simulink model "lab7"  (R2015a)
settings: Solver=ode45  StartTime=0.0  StopTime=390  RelTol=1e-3
undefined symbols (not defined in the file or in its folder): currentCFG_lab7_UB, fdesignblkfcn, gcbh, UB
libraries: dspstat3 x2, gtecHighspeedLib x1, gUSBamplib x1
settings Model: Creator=circuit  LastModifiedBy=circuit

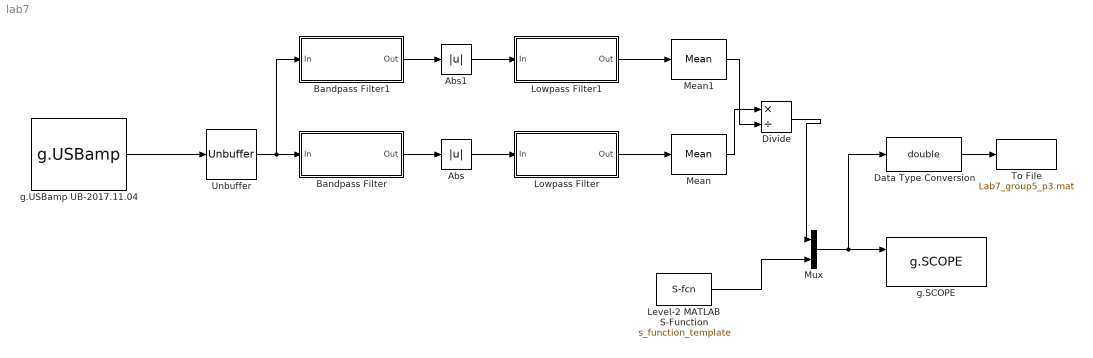
== system lab7 ==
  Abs : Abs
  Abs1 : Abs
  Bandpass Filter : Subsystem  DialogController=fdesignblkfcn  InitFcn=fdesignblkfcn(gcbh, {'InitFcn'});  mask(Bandpass Filter){}
      mask help: Design a bandpass filter
      settings: CopyFcn=fdesignblkfcn(gcbh, {'CopyFcn'});
      mask Help: helpview(mapfilelocation('dsp'), 'dspbandpassfilter');
      mask Display: disp('Bandpass');
  Bandpass Filter1 : Subsystem  DialogController=fdesignblkfcn  InitFcn=fdesignblkfcn(gcbh, {'InitFcn'});  mask(Bandpass Filter){}
      mask help: Design a bandpass filter
      settings: CopyFcn=fdesignblkfcn(gcbh, {'CopyFcn'});
      mask Help: helpview(mapfilelocation('dsp'), 'dspbandpassfilter');
      mask Display: disp('Bandpass');
  Data Type Conversion : DataTypeConversion  OutDataTypeStr=double
  Divide : Product  Inputs=*/
  Level-2 MATLAB S-Function : M-S-Function  FunctionName=s_function_template
  Lowpass Filter : Subsystem  DialogController=fdesignblkfcn  InitFcn=fdesignblkfcn(gcbh, {'InitFcn'});  mask(Lowpass Filter){}
      mask help: Design a lowpass filter
      settings: CopyFcn=fdesignblkfcn(gcbh, {'CopyFcn'});
      mask Help: helpview(mapfilelocation('dsp'), 'dsplowpassfilter');
      mask Display: disp('Lowpass')
  Lowpass Filter1 : Subsystem  DialogController=fdesignblkfcn  InitFcn=fdesignblkfcn(gcbh, {'InitFcn'});  mask(Lowpass Filter){}
      mask help: Design a lowpass filter
      settings: CopyFcn=fdesignblkfcn(gcbh, {'CopyFcn'});
      mask Help: helpview(mapfilelocation('dsp'), 'dsplowpassfilter');
      mask Display: disp('Lowpass')
  Mean : dspstat3/Mean  run=off  reset_popup=None  InputProcessing=Columns as channels (frame based)  directionMode=Each row  dimension=1  treatSBRowAsCol=off  roiEnable=off  roiType=Rectangles  roiPortion=Entire ROI  roiOutput=Individual statistics for each ROI  roiFlag=off  outputDataTypeStr=Inherit: Same as accumulator  outputLastDataTypeStr=Inherit: Same as accumulator  outputMin=[]  outputMax=[]  roundingMode=Floor  overflowMode=off
  Mean1 : dspstat3/Mean  run=off  reset_popup=None  InputProcessing=Columns as channels (frame based)  directionMode=Each row  dimension=1  treatSBRowAsCol=off  roiEnable=off  roiType=Rectangles  roiPortion=Entire ROI  roiOutput=Individual statistics for each ROI  roiFlag=off  outputDataTypeStr=Inherit: Same as accumulator  outputLastDataTypeStr=Inherit: Same as accumulator  outputMin=[]  outputMax=[]  roundingMode=Floor  overflowMode=off
  Mux : Mux  Inputs=2
  To File : ToFile  Filename=Lab7_group5_p3.mat
  Unbuffer : Unbuffer  SampleBasedProcessing=Same as frame based
  g.SCOPE : gtecHighspeedLib/g.SCOPE
  g.USBamp UB-2017.11.04 : gUSBamplib/g.USBamp  cfg=currentCFG_lab7_UB-2017.11.04.cfg  snr=UB-2017.11.04
  wires:
  g.USBamp UB-2017.11.04/1 -> Unbuffer/1
  Bandpass Filter/1(Out) -> Abs/1
  Abs/1 -> Lowpass Filter/1(In)
  Lowpass Filter/1(Out) -> Mean/1
  Unbuffer/1 -> Bandpass Filter1/1(In), Bandpass Filter/1(In)
  Mux/1 -> Data Type Conversion/1, g.SCOPE/1
  Level-2 MATLAB S-Function/1 -> Mux/2
  Data Type Conversion/1 -> To File/1
  Bandpass Filter1/1(Out) -> Abs1/1
  Abs1/1 -> Lowpass Filter1/1(In)
  Lowpass Filter1/1(Out) -> Mean1/1
  Mean/1 -> Divide/1
  Mean1/1 -> Divide/2
  Divide/1 -> Mux/1

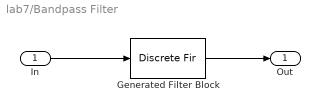
== system lab7/Bandpass Filter ==
  In : Inport
  Generated Filter Block : DiscreteFir  Tag=BlockMethodSubSystem  Coefficients=[2.7190426698472572e-18 -1.0908185879633193e-05 1.520684445102344e-05 5.9315566798347776e-05 5.800034854108737e-05 -2.0396570865799991e-05 -0.00011845969573629914 -0.00012738266702765806 -1.1513153684603061e-19 0.00017272582002327323 0.00021950102083968773 5.2546096976351294e-05 -0.00021434299056270176 -0.00033253314769670164 -0.00014434765399001844 0.0002320364222776027 0.00046047217716153568 0.00028094492726581474 -0.00021174425558163697 -0.00059175018646499215 -0.00046367795469145871 0.00013860058094126063 0.00070895386584620811 0.00068712060084153684 -2.0074243731143294e-18 -0.00079002026862442284 -0.00093727551956054834 -0.00021073549795040954 0.00081102828190988692 0.0011911833363798426 0.00049080070902079618 -0.00075036401862936866 -0.0014184160470135699 -0.00082529572189400115 0.00059369534792681842 0.001584616182718924 0.0011863604619702602 -0.00033890853760402013 -0.001656854224615913 -0.0015346613168919863 -3.7476367741136453e-18 0.0016101709367714611 0.0018234925555774587 0.00039107627928343391 -0.0014343221416268494 -0.0020053091123723812 -0.00078541019388994712 0.001139521741680656 0.002040026188317274 0.0011214198244585052 -0.00075994002810688712 -0.0019039859739218034 -0.001332349683241074 0.00035388793624190003 0.0015981839151395199 0.0013563494031183791 -1.167034324091124e-18 -0.0011542342098058455 -0.0011479613184324207 -0.00021072008592950235 0.00063667861703461156 0.00068942638733922442 0.00018647850248215282 -0.0001406111708457172 -1.8353538021468985e-17 0.00015127026108370566 -0.00021582800879737016 -0.00085849027561536707 -0.00085304304480034567 0.00030381291102699509 0.0017812926009562861 0.0019278780158680892 -1.6322403253386542e-18 -0.002626452444663831 -0.0033333696475308394 -0.00079524173104250531 0.0032266997021166946 0.0049711137239133365 0.002139805193973388 -0.0034067185066119035 -0.0066889508236326707 -0.0040345346627025658 0.0030041643873728783 0.0082906046554809907 0.0064130493527291259 -0.0018920899597823313 -0.0095523575352329977 -0.0091386778220399634 -2.4057070663414456e-18 0.010245413307559797 0.0120097217529452 0.0026693368020745799 -0.010161706291930863 -0.014773277235232266 -0.0060298998785369004 0.0091402560631568073 0.017146741075987779 0.0099111688340985694 -0.0070908496363779249 -0.018845064066358108 -0.014066562886420964 0.0040119204928050064 0.019610930916622103 0.018191355541196143 -2.0721869535670114e-17 -0.019244478222364952 -0.021948648476352237 -0.0047510042785245737 0.017629000615502922 0.025000899763098283 0.0099612960891193574 -0.014749382546861711 -0.027043678172353688 -0.015286750482589083 0.01070071066686748 0.027837877532802983 0.020348597794259786 -0.0056855921470147308 -0.02723664502279062 -0.024768224255709254 0 0.025203767584335721 0.028203363377651062 0.0059911738926469475 -0.02182117135681989 -0.030381676304823767 -0.011886427654215447 0.017284412946531557 0.031127931526122532 0.017284412946531557 -0.011886427654215447 -0.030381676304823767 -0.02182117135681989 0.0059911738926469475 0.028203363377651062 0.025203767584335721 0 -0.024768224255709254 -0.02723664502279062 -0.0056855921470147308 0.020348597794259786 0.027837877532802983 0.01070071066686748 -0.015286750482589083 -0.027043678172353688 -0.014749382546861711 0.0099612960891193574 0.025000899763098283 0.017629000615502922 -0.0047510042785245737 -0.021948648476352237 -0.019244478222364952 -2.0721869535670114e-17 0.018191355541196143 0.019610930916622103 0.0040119204928050064 -0.014066562886420964 -0.018845064066358108 -0.0070908496363779249 0.0099111688340985694 0.017146741075987779 0.0091402560631568073 -0.0060298998785369004 -0.014773277235232266 -0.010161706291930863 0.0026693368020745799 0.0120097217529452 0.010245413307559797 -2.4057070663414456e-18 -0.0091386778220399634 -0.0095523575352329977 -0.0018920899597823313 0.0064130493527291259 0.0082906046554809907 0.0030041643873728783 -0.0040345346627025658 -0.0066889508236326707 -0.0034067185066119035 0.002139805193973388 0.0049711137239133365 ...(+1777 chars)]  InputProcessing=Columns as channels (frame based)
  Out : Outport
  wires:
  In/1 -> Generated Filter Block/1
  Generated Filter Block/1 -> Out/1

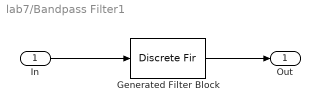
== system lab7/Bandpass Filter1 ==
  In : Inport
  Generated Filter Block : DiscreteFir  Tag=BlockMethodSubSystem  Coefficients=[9.707348092578544e-20 1.2824518125158989e-05 -5.8306790931058319e-06 -5.1094665598218423e-05 -7.8492802731727667e-05 -4.2367664329779592e-05 5.482097131385022e-05 0.00014765204534916088 0.00014937815000888054 2.5429015679797125e-05 -0.0001595529056554699 -0.00026926089870703485 -0.00019230130659421058 5.7964178583766491e-05 0.00032353356290002735 0.0003965741710622289 0.00017621481952965698 -0.00022736250597250629 -0.00053673149258709344 -0.00049328357455963464 -6.427363295049944e-05 0.00048987864431977192 0.00076644070503021353 0.00050842229855829453 -0.00017311876377014372 -0.00082671135359862178 -0.00095519480746324831 -0.00038875608868311963 0.00054067581479109029 0.0011850080422950934 0.0010301315002544447 9.9357594786191956e-05 -0.0010029701611908729 -0.0014814659125480301 -0.0009241669920431485 0.00035399274215935792 0.0014796563120018401 0.0016207814230849605 0.00060416596910270112 -0.00090975146702838806 -0.0018572633928367916 -0.0015266591337778784 -9.6846403530982854e-05 0.0014518170031156234 0.0020186674362239654 0.0011772931075391218 -0.00049868590923118352 -0.0018320762800049775 -0.0018847357273057168 -0.00063316642042513839 0.0010209135234836562 0.0019127041848916357 0.0014565250639395791 4.4516981260796249e-05 -0.0012817412050596757 -0.0016189973344774209 -0.00084311680333582319 0.00037024629768436692 0.0011232451959351355 0.0009874507299979312 0.0002613718120873643 -0.0003760669665239552 -0.00048201691806036789 -0.00019164430137375517 -4.6654510311759717e-19 -0.0002061719800045026 -0.00055788066853210009 -0.0004682876078866057 0.00035019458867089671 0.0014236909569065638 0.0017429405716484984 0.00061840975748094103 -0.0015161168971767184 -0.0031350472800490809 -0.0026733576708300949 0.00010003664327914878 0.0035274290593943084 0.0049938760860282361 0.0028746427077805323 -0.0019234721156004926 -0.0061797758615493312 -0.0064865592169339337 -0.0019074548059747262 0.0048673152971825335 0.0090257366316384285 0.0070241242451971834 -0.00050732944848053954 -0.0086646986658727911 -0.011428342065264252 -0.0060735093041513867 0.0043793020977473387 0.012765720012089456 0.01267391601250209 0.0033002521217517428 -0.0093863535439994983 -0.016407425157192592 -0.012124559431691989 0.0013123628964441651 0.014882838267642211 0.018747368095384083 0.0093775402406630435 -0.0074010241941180038 -0.01998586220395545 -0.019036220664872205 -0.0043931360632011845 0.014239599046203293 0.023728395348541657 0.016792249493582444 -0.0024436786424297165 -0.020840776199870091 -0.025249994637770418 -0.011936348557839342 0.010349152684826973 0.026126632799117634 0.023984034045009792 0.0048524476909475225 -0.01825607608125419 -0.029134564492501906 -0.019798021153016373 0.003646423927090451 0.024998853944443632 0.029214240219385793 0.013051998530556084 -0.012444839188660729 -0.02953094148171764 -0.026170897032573331 -0.004557549427059774 0.020320910329309189 0.031127886704473189 0.020320910329309189 -0.004557549427059774 -0.026170897032573331 -0.02953094148171764 -0.012444839188660729 0.013051998530556084 0.029214240219385793 0.024998853944443632 0.003646423927090451 -0.019798021153016373 -0.029134564492501906 -0.01825607608125419 0.0048524476909475225 0.023984034045009792 0.026126632799117634 0.010349152684826973 -0.011936348557839342 -0.025249994637770418 -0.020840776199870091 -0.0024436786424297165 0.016792249493582444 0.023728395348541657 0.014239599046203293 -0.0043931360632011845 -0.019036220664872205 -0.01998586220395545 -0.0074010241941180038 0.0093775402406630435 0.018747368095384083 0.014882838267642211 0.0013123628964441651 -0.012124559431691989 -0.016407425157192592 -0.0093863535439994983 0.0033002521217517428 0.01267391601250209 0.012765720012089456 0.0043793020977473387 -0.0060735093041513867 -0.011428342065264252 -0.0086646986658727911 -0.00050732944848053954 0.0070241242451971834 0.0090257366316384285 0.0048673152971825335 -0.0019074548059747262 -0.0064865592169339337 -0.0061797758615493312 -0.0019234721156004926 ...(+1818 chars)]  InputProcessing=Columns as channels (frame based)
  Out : Outport
  wires:
  In/1 -> Generated Filter Block/1
  Generated Filter Block/1 -> Out/1

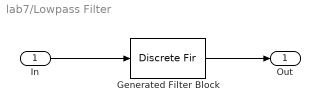
== system lab7/Lowpass Filter ==
  In : Inport
  Generated Filter Block : DiscreteFir  Tag=BlockMethodSubSystem  Coefficients=[1.4428298688351188e-20 1.45208171766696e-06 2.9191625460814213e-06 4.4049970012497788e-06 5.9133935180921881e-06 7.4482126794738371e-06 9.0133654082074441e-06 1.0612811122812577e-05 1.2250555857839479e-05 1.3930650349583523e-05 1.5657188088038609e-05 1.7434303335956318e-05 1.9266169115897482e-05 2.1156995166181424e-05 2.3111025866657028e-05 2.5132538135237749e-05 2.7225839296160136e-05 2.9395264920942651e-05 3.1645176643039415e-05 3.3979959947197383e-05 3.6404021934544024e-05 3.8921789064445974e-05 4.1537704874194934e-05 4.4256227677590849e-05 4.7081828243506648e-05 5.0018987455532009e-05 5.3072193953806083e-05 5.6245941760161995e-05 5.9544727887716448e-05 6.2973049936051491e-05 6.6535403673141706e-05 7.0236280605195109e-05 7.4080165535581819e-05 7.8071534114035083e-05 8.2214850377317441e-05 8.651456428255206e-05 9.0975109234426682e-05 9.5600899607484595e-05 0.0001003963282647219 0.00010536576407371653 0.00011051354942152003 0.0001158439977295443 0.00012136139096968262 0.00012706997718290485 0.00013297396800156886 0.00013907753617669477 0.00014538481311144461 0.00015189988640205564 0.00015862679738747154 0.00016556953870891733 0.00017273205188065983 0.00018011822487319705 0.00018773188971011259 0.00019557682007983164 0.00020365672896350919 0.00021197526628027701 0.0002205360165510704 0.00022934249658225023 0.00023839815317022907 0.00024770636082830321 0.0002572704195368833 0.00026709355251831266 0.00027717890403744435 0.00028752953722915094 0.00029814843195391652 0.00030903848268266351 0.00032020249641194509 0.00033164319061062744 0.00034336319119917153 0.00035536503056261208 0.00036765114559831707 0.0003802238757995954 0.00039308546137620996 0.00040623804141283194 0.00041968365206646155 0.00043342422480381864 0.00044746158467969812 0.00046179744865725437 0.00047643342397117616 0.00049137100653468154 0.00050661157939125266 0.00052215641121200267 0.00053800665483955796 0.00055416334587930457 0.00057062740133883758 0.00058739961831642709 0.00060448067273929083 0.00062187111815244288 0.00063957138455886719 0.00065758177731173567 0.00067590247605937262 0.00069453353374364314 0.00071347487565241133 0.00073272629852670233 0.00075228746972316328 0.00077215792643240224 0.00079233707495375701 0.0008128241900270159 0.00083361841422158797 0.00085471875738359678 0.00087612409614133886 0.00089783317346952781 0.00091984459831270988 0.00094215684526821456 0.00096476825432897483 0.00098767703068652207 0.0010108812445944334 0.0010343788312924805 0.001058167590991699 0.0010822451889205716 0.0011066091554324852 0.0011312568861745979 0.0011561856423182159 0.0011813925508507587 0.0012068746049293559 0.0012326286642960896 0.0012586514557548691 0.0012849395737099 0.0013114894807656631 0.0013382975083883106 0.0013653598576283397 0.0013926725999043852 0.0014202316778479387 0.0014480329062087722 0.0014760719728208135 0.0015043444396281973 0.0015328457437711754 0.001561571198731555 0.0015905159955372915 0.0016196752040258393 0.001649043774165836 0.0016786165374366667 0.0017083882082654166 0.0017383533855207178 0.0017685065540629331 0.0017988420863501169 0.0018293542440991598 0.0018600371800014915 0.0018908849394926963 0.001921891462575358 0.0019530505856944402 0.0019843560436644627 0.0020158014716477306 0.0020473804071828253 0.0020790862922625583 0.0021109124754605506 0.0021428522141055924 0.0021748986765028917 0.002207044944201317 0.0022392840143057066 0.0022716088018332921 0.0023040121421132637 0.0023364867932284933 0.0023690254384983803 0.0024016206890018067 0.0024342650861391263 0.0024669511042321214 0.0024996711531608206 0.0025324175810360746 0.002565182676906736 0.0025979586735003163 0.0026307377499959206 0.0026635120348282985 0.0026962736085217849 0.0027290145065529321 0.0027617267222405763 0.0027944022096621146 0.0028270328865946928 0.0028596106374800699 0.0028921273164118281 0.0029245747501436526 0.0029569447411173545 0.0029892290705093136 0.0030214195012940033 0.0030535077813232574 0.0030854856464199156 0.0031173448234844878 ...(+7462 chars)]  InputProcessing=Columns as channels (frame based)
  Out : Outport
  wires:
  In/1 -> Generated Filter Block/1
  Generated Filter Block/1 -> Out/1

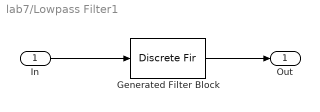
== system lab7/Lowpass Filter1 ==
  In : Inport
  Generated Filter Block : DiscreteFir  Tag=BlockMethodSubSystem  Coefficients=[1.4428298688351188e-20 1.45208171766696e-06 2.9191625460814213e-06 4.4049970012497788e-06 5.9133935180921881e-06 7.4482126794738371e-06 9.0133654082074441e-06 1.0612811122812577e-05 1.2250555857839479e-05 1.3930650349583523e-05 1.5657188088038609e-05 1.7434303335956318e-05 1.9266169115897482e-05 2.1156995166181424e-05 2.3111025866657028e-05 2.5132538135237749e-05 2.7225839296160136e-05 2.9395264920942651e-05 3.1645176643039415e-05 3.3979959947197383e-05 3.6404021934544024e-05 3.8921789064445974e-05 4.1537704874194934e-05 4.4256227677590849e-05 4.7081828243506648e-05 5.0018987455532009e-05 5.3072193953806083e-05 5.6245941760161995e-05 5.9544727887716448e-05 6.2973049936051491e-05 6.6535403673141706e-05 7.0236280605195109e-05 7.4080165535581819e-05 7.8071534114035083e-05 8.2214850377317441e-05 8.651456428255206e-05 9.0975109234426682e-05 9.5600899607484595e-05 0.0001003963282647219 0.00010536576407371653 0.00011051354942152003 0.0001158439977295443 0.00012136139096968262 0.00012706997718290485 0.00013297396800156886 0.00013907753617669477 0.00014538481311144461 0.00015189988640205564 0.00015862679738747154 0.00016556953870891733 0.00017273205188065983 0.00018011822487319705 0.00018773188971011259 0.00019557682007983164 0.00020365672896350919 0.00021197526628027701 0.0002205360165510704 0.00022934249658225023 0.00023839815317022907 0.00024770636082830321 0.0002572704195368833 0.00026709355251831266 0.00027717890403744435 0.00028752953722915094 0.00029814843195391652 0.00030903848268266351 0.00032020249641194509 0.00033164319061062744 0.00034336319119917153 0.00035536503056261208 0.00036765114559831707 0.0003802238757995954 0.00039308546137620996 0.00040623804141283194 0.00041968365206646155 0.00043342422480381864 0.00044746158467969812 0.00046179744865725437 0.00047643342397117616 0.00049137100653468154 0.00050661157939125266 0.00052215641121200267 0.00053800665483955796 0.00055416334587930457 0.00057062740133883758 0.00058739961831642709 0.00060448067273929083 0.00062187111815244288 0.00063957138455886719 0.00065758177731173567 0.00067590247605937262 0.00069453353374364314 0.00071347487565241133 0.00073272629852670233 0.00075228746972316328 0.00077215792643240224 0.00079233707495375701 0.0008128241900270159 0.00083361841422158797 0.00085471875738359678 0.00087612409614133886 0.00089783317346952781 0.00091984459831270988 0.00094215684526821456 0.00096476825432897483 0.00098767703068652207 0.0010108812445944334 0.0010343788312924805 0.001058167590991699 0.0010822451889205716 0.0011066091554324852 0.0011312568861745979 0.0011561856423182159 0.0011813925508507587 0.0012068746049293559 0.0012326286642960896 0.0012586514557548691 0.0012849395737099 0.0013114894807656631 0.0013382975083883106 0.0013653598576283397 0.0013926725999043852 0.0014202316778479387 0.0014480329062087722 0.0014760719728208135 0.0015043444396281973 0.0015328457437711754 0.001561571198731555 0.0015905159955372915 0.0016196752040258393 0.001649043774165836 0.0016786165374366667 0.0017083882082654166 0.0017383533855207178 0.0017685065540629331 0.0017988420863501169 0.0018293542440991598 0.0018600371800014915 0.0018908849394926963 0.001921891462575358 0.0019530505856944402 0.0019843560436644627 0.0020158014716477306 0.0020473804071828253 0.0020790862922625583 0.0021109124754605506 0.0021428522141055924 0.0021748986765028917 0.002207044944201317 0.0022392840143057066 0.0022716088018332921 0.0023040121421132637 0.0023364867932284933 0.0023690254384983803 0.0024016206890018067 0.0024342650861391263 0.0024669511042321214 0.0024996711531608206 0.0025324175810360746 0.002565182676906736 0.0025979586735003163 0.0026307377499959206 0.0026635120348282985 0.0026962736085217849 0.0027290145065529321 0.0027617267222405763 0.0027944022096621146 0.0028270328865946928 0.0028596106374800699 0.0028921273164118281 0.0029245747501436526 0.0029569447411173545 0.0029892290705093136 0.0030214195012940033 0.0030535077813232574 0.0030854856464199156 0.0031173448234844878 ...(+7462 chars)]  InputProcessing=Columns as channels (frame based)
  Out : Outport
  wires:
  In/1 -> Generated Filter Block/1
  Generated Filter Block/1 -> Out/1
